simulink model "srm_simulink_template"  (R2020a)
settings: Solver=ode4  StartTime=0.0  StopTime=50  FixedStep=1E-3  RelTol=1e-3
libraries: robotmaniplib x1
settings Model: Creator=fernando  LastModifiedBy=User
settings SFSimCC: CustomCodeUndefinedFunction=UseInterfaceOnly

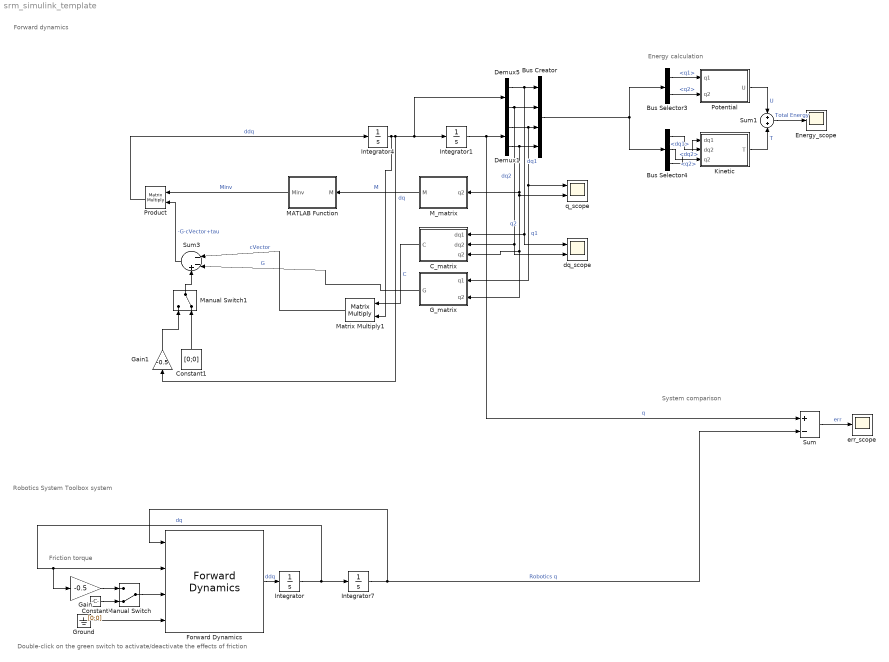
== system srm_simulink_template ==
  note: Double-click on the green switch to activate/deactivate the effects of friction
  note: Friction torque
  note: System comparison
  note: Robotics System Toolbox system
  note: Forward dynamics
  note: Energy calculation
  Bus Creator : BusCreator  Inputs=4
  Bus Selector3 : BusSelector  OutputSignals=q1,q2
  Bus Selector4 : BusSelector  OutputSignals=dq2,q2,dq1
  C_matrix : MATLAB Function  TreatAsAtomicUnit=on
  Constant : Constant  Value=[0;0]  VectorParams1D=off
  Constant1 : Constant  Value=[0;0]
  Demux1 : Demux  Outputs=2
  Demux5 : Demux  Outputs=2
  Energy_scope : Scope
  Forward Dynamics : robotmaniplib/Forward Dynamics  RigidBodyTree=twoLinkRobot  SimulateUsing=Code generation
  G_matrix : MATLAB Function  TreatAsAtomicUnit=on
  Gain : Gain  Gain=-0.5
  Gain1 : Gain  Gain=-0.5
  Ground : Ground
  Integrator : Integrator  InitialCondition=zeros(2,1)
  Integrator1 : Integrator  InitialCondition=[0 0]  WrapState=on
  Integrator4 : Integrator  InitialCondition=[0,0]
  Integrator7 : Integrator  InitialCondition=zeros(2,1)
  Kinetic : MATLAB Function  TreatAsAtomicUnit=on
  MATLAB Function : MATLAB Function  TreatAsAtomicUnit=on
  M_matrix : MATLAB Function  TreatAsAtomicUnit=on
  Manual Switch : ManualSwitch  CurrentSetting=0
  Manual Switch1 : ManualSwitch  CurrentSetting=0
  Matrix Multiply1 : Product  Multiplication=Matrix(*)  OutMin=2  OutMax=2
  Potential : MATLAB Function  TreatAsAtomicUnit=on
  Product : Product  Multiplication=Matrix(*)
  Sum : Sum  Inputs=+-
  Sum1 : Sum  Inputs=+|+
  Sum3 : Sum  Inputs=|--+
  dq_scope : Scope  NumInputPorts=2
  err_scope : Scope
  q_scope : Scope  NumInputPorts=2
  wires:
  Integrator4/1 -> Gain1/1, Demux5/1, Integrator1/1, Matrix Multiply1/2  "dq"
  Integrator1/1 -> Sum/1, Demux1/1  "q"
  Product/1 -> Integrator4/1  "ddq"
  Kinetic/1(T) -> Sum1/2  "T"
  Sum1/1 -> Energy_scope/1  "Total Energy"
  Demux5/1 -> C_matrix/1(dq1), dq_scope/1, Bus Creator/1  "dq1"
  Demux5/2 -> C_matrix/2(dq2), dq_scope/2, Bus Creator/2  "dq2"
  Demux1/1 -> G_matrix/1(q1), q_scope/1, Bus Creator/3  "q1"
  Demux1/2 -> M_matrix/1(q2), G_matrix/2(q2), C_matrix/3(q2), q_scope/2, Bus Creator/4  "q2"
  Bus Creator/1 -> Bus Selector3/1, Bus Selector4/1
  Bus Selector3/2 -> Potential/2(q2)  "<q2>"
  Bus Selector3/1 -> Potential/1(q1)  "<q1>"
  Bus Selector4/3 -> Kinetic/1(dq1)  "<dq1>"
  Bus Selector4/1 -> Kinetic/2(dq2)  "<dq2>"
  Bus Selector4/2 -> Kinetic/3(q2)  "<q2>"
  Potential/1(U) -> Sum1/1  "U"
  Forward Dynamics/1 -> Integrator/1  "ddq"
  Integrator7/1 -> Forward Dynamics/1, Sum/2  "Robotics q"
  Gain/1 -> Manual Switch/1
  Sum/1 -> err_scope/1  "err"
  Integrator/1 -> Forward Dynamics/2, Gain/1, Integrator7/1  "dq"
  Manual Switch/1 -> Forward Dynamics/3
  M_matrix/1(M) -> MATLAB Function/1(M)  "M"
  G_matrix/1(G) -> Sum3/2  "G"
  Constant/1 -> Manual Switch/2
  MATLAB Function/1(Minv) -> Product/1  "Minv"
  Sum3/1 -> Product/2  "-G-cVector+tau"
  Matrix Multiply1/1 -> Sum3/1  "cVector"
  Ground/1 -> Forward Dynamics/4
  C_matrix/1(C) -> Matrix Multiply1/1  "C"
  Gain1/1 -> Manual Switch1/1
  Constant1/1 -> Manual Switch1/2
  Manual Switch1/1 -> Sum3/3

== matlab function srm_simulink_template/M_matrix ==
  data: q2 input; M output
function M = M_matrix(q2)
%#codegen

%    This function was generated by the Symbolic Math Toolbox version 8.5.
%    04-Nov-2022 18:56:12

t2 = cos(q2);
t3 = t2./2.0;
t4 = t3+3.341666666666667e-1;
M = reshape([t2+1.668333333333333,t4,t4,3.341666666666667e-1],[2,2]);

== matlab function srm_simulink_template/G_matrix ==
  data: q1 input; G output; q2 input
function G = G_matrix(q1,q2)
%#codegen

%    This function was generated by the Symbolic Math Toolbox version 8.5.
%    04-Nov-2022 18:56:13

t2 = q1+q2;
t3 = cos(t2);
t4 = t3.*(9.81e+2./2.0e+2);
G = [t4+cos(q1).*1.4715e+1;t4];

== matlab function srm_simulink_template/Kinetic ==
  data: dq1 input; T output; dq2 input; q2 input
function T = Kinetic(dq1,dq2,q2)
%#codegen

%    This function was generated by the Symbolic Math Toolbox version 8.5.
%    04-Nov-2022 18:56:13

t2 = cos(q2);
t3 = t2./2.0;
t4 = t3+3.341666666666667e-1;
T = dq2.*(dq2.*1.670833333333333e-1+(dq1.*t4)./2.0)+dq1.*((dq2.*t4)./2.0+(dq1.*(t2+1.668333333333333))./2.0);

== matlab function srm_simulink_template/Potential ==
  data: q1 input; U output; q2 input
function U = Potential(q1,q2)
%#codegen

%    This function was generated by the Symbolic Math Toolbox version 8.5.
%    04-Nov-2022 18:56:13

U = sin(q1+q2).*(9.81e+2./2.0e+2)+sin(q1).*1.4715e+1;

== matlab function srm_simulink_template/MATLAB Function ==
  data: M input size=[2 2]; Minv output size=[2 2]
function Minv = fcn(M)
Minv = inv(M);

== matlab function srm_simulink_template/C_matrix ==
  data: dq1 input; C output; dq2 input; q2 input
function C = C_matrix(dq1,dq2,q2)
%#codegen

%    This function was generated by the Symbolic Math Toolbox version 8.5.
%    04-Nov-2022 18:56:12

t2 = sin(q2);
t3 = (dq1.*t2)./2.0;
t4 = (dq2.*t2)./2.0;
t5 = -t4;
C = reshape([t5,t3,-t3+t5,0.0],[2,2]);
